simulink model "fichier_simulink"  (R2020a)
settings: Solver=VariableStepAuto  StartTime=0.0  StopTime=10.0  RelTol=1e-3
values from neighbouring files (symbols this model uses):
  a = H/2    (= 0.5)    [Preparation.m]    (also in matlab.m)
  k1 = 0.5    [Preparation.m]    (also in matlab.m)
  Km = 42.8    [matlab.m]
  Ps = 1.58    [matlab.m]
  Rr = 1/9    (= 0.111111111111)    [matlab.m]
  Sr = 7.25    [matlab.m]
  tau = 0.214    [Preparation.m]    (also in matlab.m)
settings Model: Creator=predon  LastModifiedBy=predon

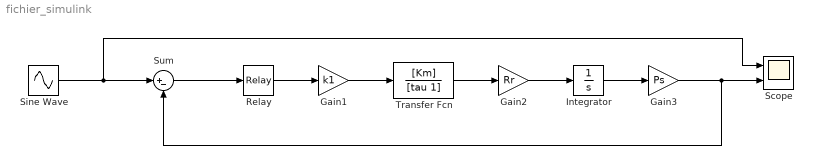
== system fichier_simulink ==
  Gain1 : Gain  Gain=k1
  Gain2 : Gain  Gain=Rr
  Gain3 : Gain  Gain=Ps
  Integrator : Integrator
  Relay : Relay  OnSwitchValue=a  OffSwitchValue=-a  OnOutputValue=Sr  OffOutputValue=-Sr
  Scope : Scope  NumInputPorts=2
  Sine Wave : Sin  Amplitude=1.5  Frequency=314.1593  SampleTime=0
  Sum : Sum  Inputs=|+-
  Transfer Fcn : TransferFcn  Numerator=[Km]  Denominator=[tau 1]
  wires:
  Sum/1 -> Relay/1
  Relay/1 -> Gain1/1
  Gain1/1 -> Transfer Fcn/1
  Transfer Fcn/1 -> Gain2/1
  Gain2/1 -> Integrator/1
  Integrator/1 -> Gain3/1
  Gain3/1 -> Sum/2, Scope/2
  Sine Wave/1 -> Scope/1, Sum/1
